simulink model "MidEval1Mux3"  (R2022b)
settings: Solver=VariableStepAuto  StartTime=0.0  StopTime=0.5  MaxStep=1e-1  RelTol=1e-4
model workspace (MAT data in the model file):
  DataStore = Simulink.Parameter
  DataStore.Value = [1 0 0 1 0 0 0 1 1 0 0 1 ... (2240 elements, 2240x1)]
  DataStore.DataType = 'auto'
  DataStore.Complexity = 'real'
  DataStore.Dimensions = [2240 1]
  Freq = Simulink.Parameter
  Freq.Value = 2000
  Freq.DataType = 'auto'
  Freq.Complexity = 'real'
  Freq.Dimensions = [1 1]
  Freq2 = Simulink.Parameter
  Freq2.Value = 6000000
  Freq2.DataType = 'auto'
  Freq2.Complexity = 'real'
  Freq2.Dimensions = [1 1]
  Freq3 = Simulink.Parameter
  Freq3.Value = 3000000
  Freq3.DataType = 'auto'
  Freq3.Complexity = 'real'
  Freq3.Dimensions = [1 1]
  Freq4 = Simulink.Parameter
  Freq4.Value = 10000000
  Freq4.DataType = 'auto'
  Freq4.Complexity = 'real'
  Freq4.Dimensions = [1 1]
  fsr = 20
libraries: commdigbbndam3 x5, commrandsrc3 x3, hdlsllib x2, dspfdesign x2, commfilt2 x2, commchan3 x1, eeGeneralControl x1
settings Model: Creator=Ceribro  LastModifiedBy=Ceribro

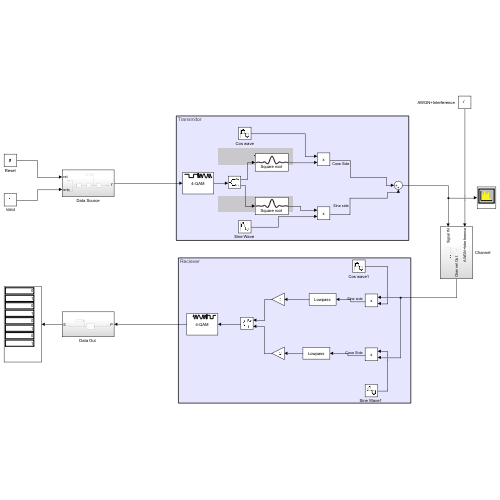
[thumbnail: Simulink's stored preview of the top-level diagram]
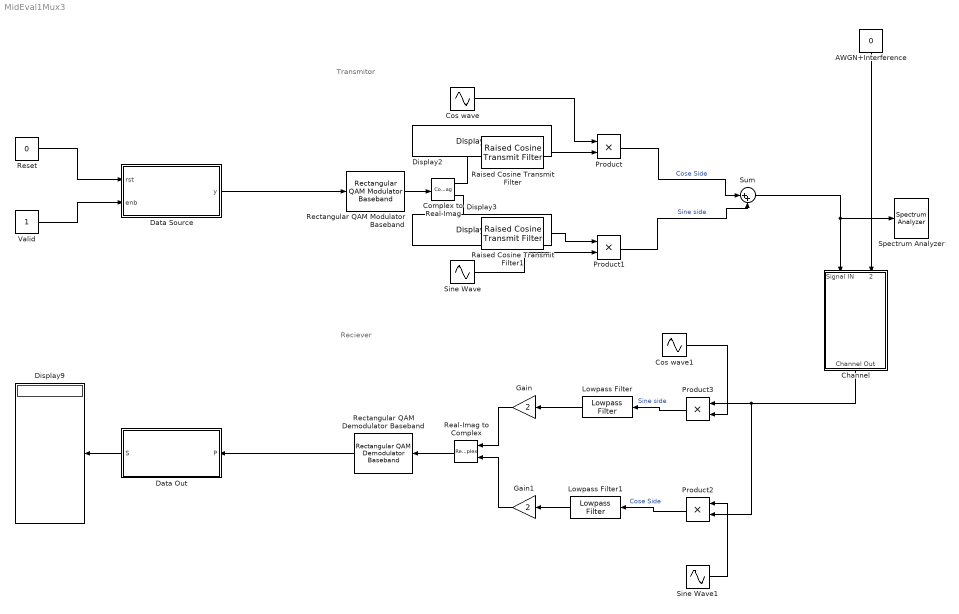
== system MidEval1Mux3 ==
  note: Reciever
  note: Transmitor
  "AWGN+Interference " : Constant  Value=0
  Channel : Subsystem
  Complex to Real-Imag : ComplexToRealImag
  Cos wave : Sin  Frequency=2*pi*Freq  Phase=pi/2  SampleTime=1/44100  VectorParams1D=off
  Cos wave1 : Sin  Frequency=2*pi*Freq  Phase=pi/2  SampleTime=1/44100  VectorParams1D=off
  "Data Out " : Subsystem
  Data Source : Subsystem
  Display2 : DisplayBlock  LabelPosition=Hide  Transparency=1
  Display3 : DisplayBlock  LabelPosition=Hide  Transparency=1
  Display9 : Display
  Gain : Gain  Gain=2
  Gain1 : Gain  Gain=2
  Lowpass Filter : dspfdesign/Lowpass Filter  FilterType=FIR  DesignForMinimumOrder=on  FilterOrder=50  PassbandFrequency=0.25e3  StopbandFrequency=0.5e3  PassbandRipple=0.1  StopbandAttenuation=150  InheritSampleRate=off  SampleRate=44100  SimulateUsing=Interpreted execution  roundingMode=Floor  coeffsDataTypeStr=fixdt(1,16)
  Lowpass Filter1 : dspfdesign/Lowpass Filter  FilterType=FIR  DesignForMinimumOrder=on  FilterOrder=50  PassbandFrequency=0.5e3  StopbandFrequency=1e3  PassbandRipple=0.1  StopbandAttenuation=80  InheritSampleRate=off  SampleRate=44100  SimulateUsing=Interpreted execution  roundingMode=Floor  coeffsDataTypeStr=fixdt(1,16)
  Product{,1..3} (4 alike) : Product
  Raised Cosine Transmit Filter : commfilt2/Raised Cosine Transmit Filter  filtType=Square root  R=0.2  filtSpan=10  N=8  filterGain=1  InputProcessing=Columns as channels (frame based)  RateOptions=Enforce single-rate processing  framing=Mute  checkCoeff=off  variableName=rcTxFilt  checkGain=Normalized  sampMode=Mute  saveAsFlag=0  currentFiltSpan=10  D=(10)/2  launchFVT=on  roundingMode=Floor  overflowMode=off  coeffDataTypeStr=Inherit: Same word length as input  coeffMin=[]  coeffMax=[]  coeffLastDataTypeStr=Inherit: Same word length as input  outputDataTypeStr=Inherit: Same as accumulator  outputMin=[]  outputMax=[]  outputLastDataTypeStr=Inherit: Same as accumulator
  Raised Cosine Transmit Filter1 : commfilt2/Raised Cosine Transmit Filter  filtType=Square root  R=0.2  filtSpan=10  N=8  filterGain=1  InputProcessing=Columns as channels (frame based)  RateOptions=Enforce single-rate processing  framing=Mute  checkCoeff=off  variableName=rcTxFilt1  checkGain=Normalized  sampMode=Mute  saveAsFlag=0  currentFiltSpan=10  D=(10)/2  launchFVT=on  roundingMode=Floor  overflowMode=off  coeffDataTypeStr=Inherit: Same word length as input  coeffMin=[]  coeffMax=[]  coeffLastDataTypeStr=Inherit: Same word length as input  outputDataTypeStr=Inherit: Same as accumulator  outputMin=[]  outputMax=[]  outputLastDataTypeStr=Inherit: Same as accumulator
  Real-Imag to Complex : RealImagToComplex
  Rectangular QAM Demodulator Baseband : commdigbbndam3/Rectangular QAM Demodulator Baseband  M=4  OutType=Bit  DecType=Hard decision  VarSource=Dialog  Variance=1  Dec=Binary  Mapping=[0:15]  PowType=Min. distance between symbols  MinDist=2  AvgPow=1  PeakPow=1  Ph=0  outDtype1=int8  outDtype2=Inherit via internal rule  derotateFactorWordLen=16  derotateFactorDataTypeStr=Inherit: Same word length as input  derotateFactorLastDataTypeStr=Inherit: Same word length as input  denormFactorWordLen=16  denormFactorDataTypeStr=Inherit: Same word length as input  denormFactorLastDataTypeStr=Inherit: Same word length as input  prodOutWordLen=32  prodOutOverflowMode=Wrap  prodOutRoundingMode=Floor  prodOutOvFlMode=off  prodOutOvFlModeLastStrValue=off  sumWordLen=32
      settings: LibrarySourceBlock=|
      | commhdldigbbndam/Rectangular QAM
      | Demodulator
      | Baseband
  Rectangular QAM Modulator Baseband : commdigbbndam3/Rectangular QAM Modulator Baseband  M=4  InType=Bit  Enc=Binary  Mapping=[0:15]  PowType=Min. distance between symbols  MinDist=2  AvgPow=1  PeakPow=1  Ph=0  outDtype=Fixed-point  outWordLen=16  outUDDataType=sfix(16)  outFracLenMode=User-defined  outFracLen=0  outDataTypeStr=fixdt(1,16,0)  outLastDataTypeStr=fixdt(1,16,0)
      settings: LibrarySourceBlock=|
      | commhdldigbbndam/Rectangular QAM
      | Modulator
      | Baseband
  Reset : Constant  Value=0  OutDataTypeStr=boolean
  "Sine Wave " : Sin  Frequency=2*pi*Freq  SampleTime=1/44100  VectorParams1D=off
  "Sine Wave1 " : Sin  Frequency=2*pi*Freq  SampleTime=1/44100
  Spectrum Analyzer : SpectrumAnalyzer
  Sum : Sum  Inputs=|++
  Valid : Constant  OutDataTypeStr=boolean  SampleTime=1/44100
  wires:
  Reset/1 -> Data Source/1(rst)
  Valid/1 -> Data Source/2(enb)
  Complex to Real-Imag/2 -> Raised Cosine Transmit Filter1/1
  Rectangular QAM Modulator Baseband/1 -> Complex to Real-Imag/1
  Complex to Real-Imag/1 -> Raised Cosine Transmit Filter/1
  Data Source/1(y) -> Rectangular QAM Modulator Baseband/1
  Cos wave/1 -> Product/1
  "Sine Wave "/1 -> Product1/2
  Product/1 -> Sum/1  "Cose Side"
  Product1/1 -> Sum/2  "Sine side"
  Cos wave1/1 -> Product3/2
  Product2/1 -> Lowpass Filter1/1  "Cose Side"
  Lowpass Filter/1 -> Gain/1
  Gain1/1 -> Real-Imag to Complex/2
  Lowpass Filter1/1 -> Gain1/1
  Real-Imag to Complex/1 -> Rectangular QAM Demodulator Baseband/1
  Product3/1 -> Lowpass Filter/1  "Sine side"
  Gain/1 -> Real-Imag to Complex/1
  "Sine Wave1 "/1 -> Product2/1
  Rectangular QAM Demodulator Baseband/1 -> "Data Out "/1(P)
  "Data Out "/1(S) -> Display9/1
  "AWGN+Interference "/1 -> Channel/2(AWGN+Interference)
  Sum/1 -> Channel/1(Signal IN), Spectrum Analyzer/1
  Channel/1(Channel Out) -> Product2/2, Product3/1
  Raised Cosine Transmit Filter/1 -> Product/2
  Raised Cosine Transmit Filter1/1 -> Product1/1

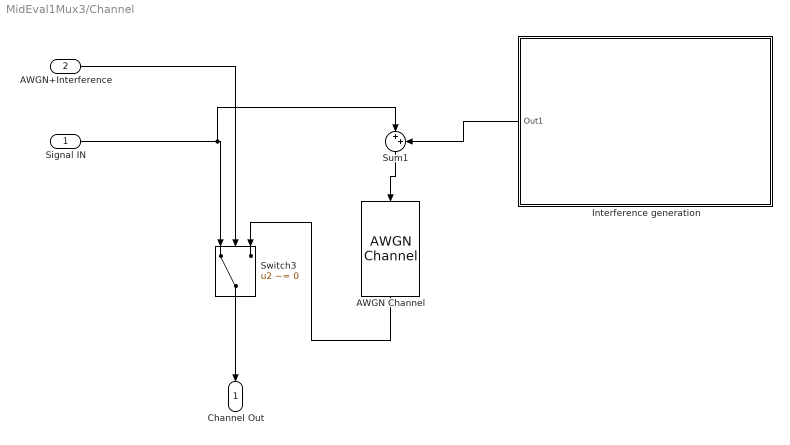
== system MidEval1Mux3/Channel ==
  Signal IN : Inport
  AWGN+Interference : Inport  Port=2
  AWGN Channel : commchan3/AWGN Channel  InputProcessing=Columns as channels (frame based)  seed=67  noiseMode="Signal to noise ratio  (Eb/No)"  EbNodB=10  EsNodB=10  SNRdB=10  bitsPerSym=1  Ps=1  Tsym=1  variance=1
  Interference generation : Subsystem
  Sum1 : Sum  Inputs=|++
  Switch3 : Switch  Criteria=u2 ~= 0  Threshold=1  SaturateOnIntegerOverflow=off  InputSameDT=off
  Channel Out : Outport
  wires:
  Signal IN/1 -> Sum1/1, Switch3/1
  AWGN+Interference/1 -> Switch3/2
  Switch3/1 -> Channel Out/1
  Interference generation/1(Out1) -> Sum1/2
  Sum1/1 -> AWGN Channel/1
  AWGN Channel/1 -> Switch3/3

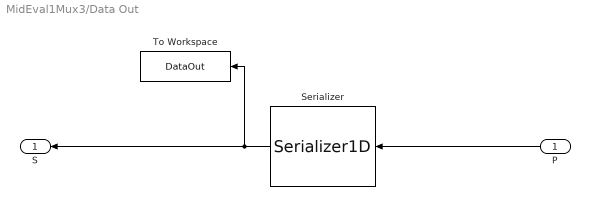
== system MidEval1Mux3/Data Out  ==
  P : Inport
  Serializer : hdlsllib/HDL Operations/Serializer1D  Ratio=2  IdleCycles=0  validIn=off  startOut=off  validOut=off  inputDataDimensions=-1  inputSampleTime=-1  inputSignalType=auto
  To Workspace : ToWorkspace  VariableName=DataOut  SampleTime=-1
      settings: Save2DSignal=2-D array (concatenate along first dimension)
  S : Outport
  wires:
  Serializer/1 -> S/1, To Workspace/1
  P/1 -> Serializer/1

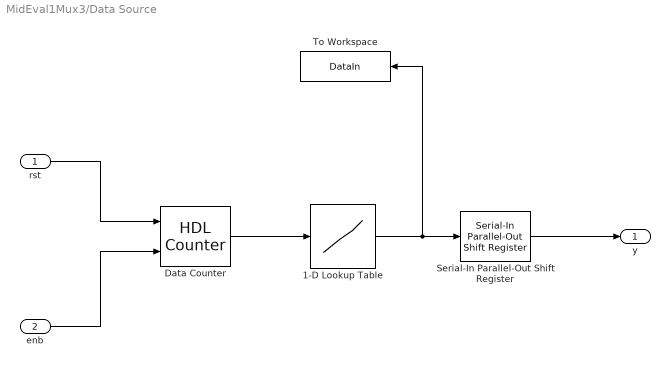
== system MidEval1Mux3/Data Source ==
  rst : Inport
  enb : Inport  Port=2
  1-D Lookup Table : Lookup_n-D  NumberOfTableDimensions=1  LookupTableObject=''  BreakpointsForDimension1=0:length(DataStore)-1  BreakpointsForDimension1FirstPoint=10  BreakpointsForDimension2FirstPoint=10  BreakpointsForDimension1Spacing=12  BreakpointsForDimension2Spacing=12  IndexSearchMethod=Evenly spaced points  Table=DataStore  TableDataTypeStr=int8  InterpMethod=Flat  DiagnosticForOutOfRangeInput=Error  InternalRulePriority=Speed  OutDataTypeStr=int8  RndMeth=Simplest
  Data Counter : hdlsllib/Sources/HDL Counter  CountType=Count limited  CountInit=0  CountStep=1  CountMax=length(DataStore)-1  CountFromType=Specify  CountFrom=0  CountResetPort=on  CountLoadPort=off  CountEnbPort=on  CountDirPort=off  CountHitOutputPort=off  CountDataType=Unsigned  CountWordLen=nextpow2(length(DataStore)-1)  CountFracLen=0  CountSampTime=1
  Serial-In Parallel-Out Shift Register : eeGeneralControl/Serial-In Parallel-Out Shift Register  N=2  IC=0  Ts=1
      settings: LibrarySourceBlock=|
      | ee_sl_lib/General Control/Serial-In Parallel-Out
      | Shift Register
  To Workspace : ToWorkspace  VariableName=DataIn  SampleTime=-1
      settings: Save2DSignal=2-D array (concatenate along first dimension)
  y : Outport
  wires:
  rst/1 -> Data Counter/1
  Data Counter/1 -> 1-D Lookup Table/1
  enb/1 -> Data Counter/2
  1-D Lookup Table/1 -> To Workspace/1, Serial-In Parallel-Out Shift Register/1
  Serial-In Parallel-Out Shift Register/1 -> y/1

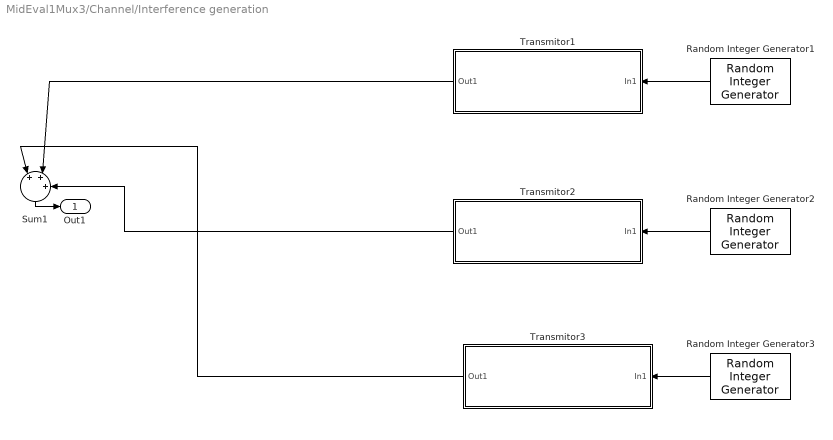
== system MidEval1Mux3/Channel/Interference generation ==
  Random Integer Generator1 : commrandsrc3/Random Integer Generator  SetSize=64  SeedSource=Auto  Seed=0  SampleTime=0.1  SamplesPerFrame=1  OutputDataType=double  SimulateUsing=Interpreted execution
  Random Integer Generator2 : commrandsrc3/Random Integer Generator  SetSize=64  SeedSource=Auto  Seed=0  SampleTime=0.1  SamplesPerFrame=1  OutputDataType=double  SimulateUsing=Interpreted execution
  Random Integer Generator3 : commrandsrc3/Random Integer Generator  SetSize=64  SeedSource=Auto  Seed=0  SampleTime=0.1  SamplesPerFrame=1  OutputDataType=double  SimulateUsing=Interpreted execution
  Sum1 : Sum  Inputs=|+++
  Transmitor1 : Subsystem
  Transmitor2 : Subsystem
  Transmitor3 : Subsystem
  Out1 : Outport
  wires:
  Random Integer Generator3/1 -> Transmitor3/1(In1)
  Transmitor3/1(Out1) -> Sum1/1
  Random Integer Generator1/1 -> Transmitor1/1(In1)
  Sum1/1 -> Out1/1
  Transmitor1/1(Out1) -> Sum1/2
  Random Integer Generator2/1 -> Transmitor2/1(In1)
  Transmitor2/1(Out1) -> Sum1/3

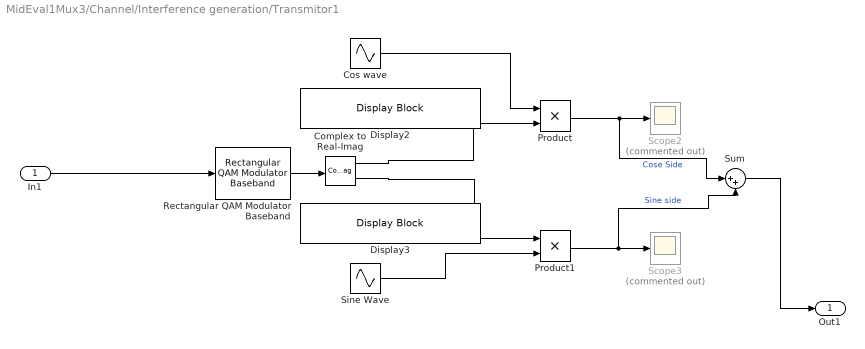
== system MidEval1Mux3/Channel/Interference generation/Transmitor1 ==
  In1 : Inport
  Complex to Real-Imag : ComplexToRealImag
  Cos wave : Sin  Frequency=2*pi*Freq2  Phase=pi/2  SampleTime=1/44100  VectorParams1D=off
  Display2 : DisplayBlock  LabelPosition=Hide  Transparency=1
  Display3 : DisplayBlock  LabelPosition=Hide  Transparency=1
  Product : Product
  Product1 : Product
  Rectangular QAM Modulator Baseband : commdigbbndam3/Rectangular QAM Modulator Baseband  M=64  InType=Integer  Enc=Binary  Mapping=[0:15]  PowType=Min. distance between symbols  MinDist=2  AvgPow=1  PeakPow=1  Ph=0  outDtype=Fixed-point  outWordLen=16  outUDDataType=sfix(16)  outFracLenMode=User-defined  outFracLen=0  outDataTypeStr=fixdt(1,16,0)  outLastDataTypeStr=fixdt(1,16,0)
      settings: LibrarySourceBlock=|
      | commhdldigbbndam/Rectangular QAM
      | Modulator
      | Baseband
  Scope2 : Scope  Commented=on
  Scope3 : Scope  Commented=on
  "Sine Wave " : Sin  Frequency=2*pi*Freq2  SampleTime=1/44100  VectorParams1D=off
  Sum : Sum  Inputs=|++
  Out1 : Outport
  wires:
  Product/1 -> Scope2/1, Sum/1  "Cose Side"
  Rectangular QAM Modulator Baseband/1 -> Complex to Real-Imag/1
  Product1/1 -> Scope3/1, Sum/2  "Sine side"
  Complex to Real-Imag/1 -> Product/2
  "Sine Wave "/1 -> Product1/2
  Cos wave/1 -> Product/1
  Complex to Real-Imag/2 -> Product1/1
  In1/1 -> Rectangular QAM Modulator Baseband/1
  Sum/1 -> Out1/1

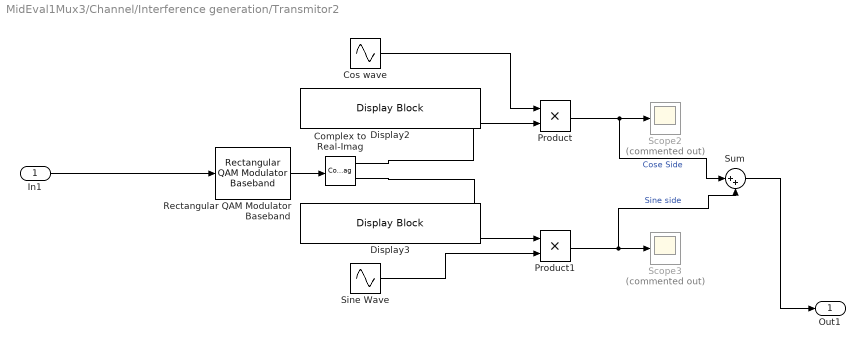
== system MidEval1Mux3/Channel/Interference generation/Transmitor2 ==
  In1 : Inport
  Complex to Real-Imag : ComplexToRealImag
  Cos wave : Sin  Frequency=2*pi*Freq3  Phase=pi/2  SampleTime=1/44100  VectorParams1D=off
  Display2 : DisplayBlock  LabelPosition=Hide  Transparency=1
  Display3 : DisplayBlock  LabelPosition=Hide  Transparency=1
  Product : Product
  Product1 : Product
  Rectangular QAM Modulator Baseband : commdigbbndam3/Rectangular QAM Modulator Baseband  M=64  InType=Integer  Enc=Binary  Mapping=[0:15]  PowType=Min. distance between symbols  MinDist=2  AvgPow=1  PeakPow=1  Ph=0  outDtype=Fixed-point  outWordLen=16  outUDDataType=sfix(16)  outFracLenMode=User-defined  outFracLen=0  outDataTypeStr=fixdt(1,16,0)  outLastDataTypeStr=fixdt(1,16,0)
      settings: LibrarySourceBlock=|
      | commhdldigbbndam/Rectangular QAM
      | Modulator
      | Baseband
  Scope2 : Scope  Commented=on
  Scope3 : Scope  Commented=on
  "Sine Wave " : Sin  Frequency=2*pi*Freq3  SampleTime=1/44100  VectorParams1D=off
  Sum : Sum  Inputs=|++
  Out1 : Outport
  wires:
  Product/1 -> Scope2/1, Sum/1  "Cose Side"
  Rectangular QAM Modulator Baseband/1 -> Complex to Real-Imag/1
  Product1/1 -> Scope3/1, Sum/2  "Sine side"
  Complex to Real-Imag/1 -> Product/2
  "Sine Wave "/1 -> Product1/2
  Cos wave/1 -> Product/1
  Complex to Real-Imag/2 -> Product1/1
  In1/1 -> Rectangular QAM Modulator Baseband/1
  Sum/1 -> Out1/1

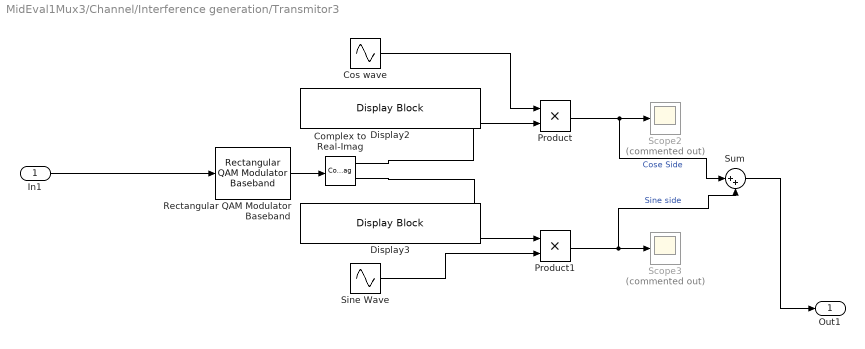
== system MidEval1Mux3/Channel/Interference generation/Transmitor3 ==
  In1 : Inport
  Complex to Real-Imag : ComplexToRealImag
  Cos wave : Sin  Frequency=2*pi*Freq4  Phase=pi/2  SampleTime=1/44100  VectorParams1D=off
  Display2 : DisplayBlock  LabelPosition=Hide  Transparency=1
  Display3 : DisplayBlock  LabelPosition=Hide  Transparency=1
  Product : Product
  Product1 : Product
  Rectangular QAM Modulator Baseband : commdigbbndam3/Rectangular QAM Modulator Baseband  M=64  InType=Integer  Enc=Binary  Mapping=[0:15]  PowType=Min. distance between symbols  MinDist=2  AvgPow=1  PeakPow=1  Ph=0  outDtype=Fixed-point  outWordLen=16  outUDDataType=sfix(16)  outFracLenMode=User-defined  outFracLen=0  outDataTypeStr=fixdt(1,16,0)  outLastDataTypeStr=fixdt(1,16,0)
      settings: LibrarySourceBlock=|
      | commhdldigbbndam/Rectangular QAM
      | Modulator
      | Baseband
  Scope2 : Scope  Commented=on
  Scope3 : Scope  Commented=on
  "Sine Wave " : Sin  Frequency=2*pi*Freq4  SampleTime=1/44100  VectorParams1D=off
  Sum : Sum  Inputs=|++
  Out1 : Outport
  wires:
  Product/1 -> Scope2/1, Sum/1  "Cose Side"
  Rectangular QAM Modulator Baseband/1 -> Complex to Real-Imag/1
  Product1/1 -> Scope3/1, Sum/2  "Sine side"
  Complex to Real-Imag/1 -> Product/2
  "Sine Wave "/1 -> Product1/2
  Cos wave/1 -> Product/1
  Complex to Real-Imag/2 -> Product1/1
  In1/1 -> Rectangular QAM Modulator Baseband/1
  Sum/1 -> Out1/1
